simulink library "SimscapeCustomComponents_lib"  (R2025b)
settings: Solver=VariableStepAuto  StartTime=0.0  StopTime=10.0  RelTol=1e-3
undefined symbols (not defined in the file or in its folder): base, baseVdc, capacity, DiscIntNeverNeededParam, ee_sli_rtmsupport, filterInductance, freqeuncy, frequency, gcbh, gflInverter, gfmInverter, iMaxPU, Inertia, initialSOC, plantRating, solar, Ts, ups, Vac, windSystem, windTurbine
libraries: fl_lib x397, nesl_utility x171, eeGeneralControl x85, ee_lib x82, simulink x72, datacenter_lib x68, eeTransforms x38, slpidlib x24, buildingEnergy_lib x20, SimscapeFluids_lib x17, eeSinusoidalMeasurementV2 x8, eePwmGenerator x8
(part 6 of 24)

== system SimscapeCustomComponents_lib/Datacenter/Facilities/Solid State Transformer ==
  note: Cascaded H-Bridge modules with DAB
  note: DAB Control
  note: Rectifier Control
  Constant1 : Constant  Value=dcBusVoltage
  Constant2 : Constant  Value=0
  Converters : Subsystem
      settings: PortSchema="{\"entries\":[{\"content\":{\"sides\":[{\"content\":{\"connectorIds\":[\"In1\",\"In2\",\"LConn1\"]},\"type\":\"ConnectorPlacement.EquallySpacedRectSide\",\"uuid\":\"3c50ecae-d327-4517-ac35-d4ccad8214d6\"},{\"content\":{\"connectorIds\":[\"RConn1\",\"RConn2\",\"Out1\",\"Out2\"],\"side\":\"RIGHT\"},\"type\":\"ConnectorPlacement.EquallySpacedRectSide\",\"uuid\":\"ce483151-8cc4-4e89-a036-44eb982feae5\"},{\"content\":{\"side\":\"TOP\"},\"type\":\"ConnectorPlacement.EquallySpacedRectSide\",\"uuid\":\"39146706-ffb9-4bd3-97cb-72551c78d2ac\"}]},\"type\":\"ConnectorPlacement.EquallySpacedConnector\",\"uuid\":\"8cf16702-94fc-4b9b-91c9-b502d0239b3b\"}],\"packageUris\":[\"http://schema.mathworks.com/mf0/Connector/R2020b\"],\"version\":\"1.0\"}"
  DAB Controller : Subsystem
  DC Voltage Balancing : Subsystem
  Filter & AC measurements : Subsystem
  PFC Rectifier Controller : Subsystem  LoadFcn=%ee_sli_rtmsupport( 'loadfcn', gcbh );  mask(PFC Rectifier Controller (Three-Phase)){Freq=60, L=0.01, BaseImpedance=9.522, KpPLL=15, KiPLL=100, Ts=5e-05, KpVoltage=18, KiVoltage=500, KdVoltage=0, NdVoltage=100, BaseVdc=4400, VoltControlUpperLimit=1, VoltControlLowerLimit=-1, KpdCurrent=10, KidCurrent=200, KddCurrent=0, IdControlUpperLimit=1, IdControlLowerLimit=-1, KpqCurrent=10, KiqCurrent=200, KdqCurrent=0, NdCurrent=100, IqControlUpperLimit=1, IqControlLowerLimit=-1}
      mask prompts: Freq "physmod:ee:library:comments:control:eeConverterControllers:SystemFrequencyHz_MP"; L "physmod:ee:library:comments:control:eeConverterControllers:ACFilterInductanceH_MP"; BaseImpedance "physmod:ee:library:comments:control:eeConverterControllers:ACSideBaseImpedanceOhm_MP"; KpPLL "physmod:ee:library:comments:control:eeConverterControllers:PLLProportionalGain_MP"; KiPLL "physmod:ee:library:comments:control:eeConverterControllers:PLLIntegralGain_MP"; Ts "physmod:ee:library:comments:control:eeConverterControllers:SampleTime1ForInherited_MP"; KpVoltage "physmod:ee:library:comments:control:eeConverterControllers:ProportionalGain_MP"; KiVoltage "physmod:ee:library:comments:control:eeConverterControllers:IntegralGain_MP"; KdVoltage "physmod:ee:library:comments:control:eeConverterControllers:DerivativeGain_MP"; NdVoltage "physmod:ee:library:comments:control:eeConverterControllers:DerivativeControllerFilterCoefficientN_MP"; BaseVdc "physmod:ee:library:comments:control:eeConverterControllers:DCBusBaseVoltageV_MP"; VoltControlUpperLimit "physmod:ee:library:comments:control:eeConverterControllers:ControllerOutputUpperLimitpu_MP"; VoltControlLowerLimit "physmod:ee:library:comments:control:eeConverterControllers:ControllerOutputLowerLimitpu_MP"; KpdCurrent "physmod:ee:library:comments:control:eeConverterControllers:IdProportionalGain_MP"; KidCurrent "physmod:ee:library:comments:control:eeConverterControllers:IdIntegralGain_MP"; KddCurrent "physmod:ee:library:comments:control:eeConverterControllers:IdDerivativeGain_MP"; IdControlUpperLimit "physmod:ee:library:comments:control:eeConverterControllers:IdControllerOutputUpperLimitpu_MP"; IdControlLowerLimit "physmod:ee:library:comments:control:eeConverterControllers:IdControllerOutputLowerLimitpu_MP"; KpqCurrent "physmod:ee:library:comments:control:eeConverterControllers:IqProportionalGain_MP"; KiqCurrent "physmod:ee:library:comments:control:eeConverterControllers:IqIntegralGain_MP"; KdqCurrent "physmod:ee:library:comments:control:eeConverterControllers:IqDerivativeGain_MP"; NdCurrent "physmod:ee:library:comments:control:eeConverterControllers:DerivativeCurrentControllerFilterCoefficientN_MP"; IqControlUpperLimit "physmod:ee:library:comments:control:eeConverterControllers:IqControllerOutputUpperLimitpu_MP"; IqControlLowerLimit "physmod:ee:library:comments:control:eeConverterControllers:IqControllerOutputLowerLimitpu_MP"
      mask help: physmod:ee:library:comments:control:eeConverterControllers:PFCRectifierController_MD
      mask init:
      | ee.mask.initializePFCController(gcb,Ts, Freq, L,BaseImpedance,KpPLL,KiPLL,KpVoltage,KiVoltage,KdVoltage,BaseVdc, NdVoltage,VoltControlUpperLimit,VoltControlLowerLimit,KpdCurrent, KidCurrent, KddCurrent, NdCurrent, IdControlUpperLimit, IdControlLowerLimit, KpqCurrent, KiqCurrent, KdqCurrent, IqControlUpperLimit, IqControlLowerLimit);
      settings: CopyFcn=%ee_sli_rtmsupport( 'copyfcn', gcbh );  DeleteFcn=ee_sli_rtmsupport( 'deletefcn', gcbh );  ModelCloseFcn=ee_sli_rtmsupport( 'modelclosefcn', gcbh );  PostSaveFcn=ee_sli_rtmsupport( 'postsavefcn', gcbh );  PreCopyFcn=ee_sli_rtmsupport( 'precopyfcn', gcbh );  OpenFcn=ee_sli_rtmsupport( 'openfcn', gcbh );  CloseFcn=%ee_sli_rtmsupport( 'closefcn', gcbh );  PreDeleteFcn=ee_sli_rtmsupport( 'predeletefcn', gcbh );
      mask Help: web(nesl_help(gcbh))
      mask DialogControl GeneralTabVal Prompt: physmod:ee:library:comments:control:eeConverterControllers:tab_General
      mask DialogControl Freq Prompt: System frequency (Hz)
      mask DialogControl L Prompt: AC filter inductance (H)
      mask DialogControl BaseImpedance Prompt: AC side base impedance (Ohm)
      mask DialogControl KpPLL Prompt: PLL proportional gain
      mask DialogControl KiPLL Prompt: PLL integral gain
      mask DialogControl Ts Prompt: Sample time (-1 for inherited)
      mask DialogControl VoltageControl Prompt: physmod:ee:library:comments:control:eeConverterControllers:tab_VoltageController
      mask DialogControl KpVoltage Prompt: Proportional gain
      mask DialogControl KiVoltage Prompt: Integral gain
      mask DialogControl KdVoltage Prompt: Derivative gain
      mask DialogControl NdVoltage Prompt: Derivative controller filter coefficient (N)
      mask DialogControl BaseVdc Prompt: DC bus base voltage (V)
      mask DialogControl VoltControlUpperLimit Prompt: Controller output upper limit (pu)
      mask DialogControl VoltControlLowerLimit Prompt: Controller output lower limit (pu)
      mask DialogControl CurrentControl Prompt: physmod:ee:library:comments:control:eeConverterControllers:tab_CurrentController
      mask DialogControl KpdCurrent Prompt: Id proportional gain
      mask DialogControl KidCurrent Prompt: Id integral gain
      mask DialogControl KddCurrent Prompt: Id derivative gain
      mask DialogControl IdControlUpperLimit Prompt: Id controller output upper limit (pu)
      mask DialogControl IdControlLowerLimit Prompt: Id controller output lower limit (pu)
      mask DialogControl KpqCurrent Prompt: Iq proportional gain
      mask DialogControl KiqCurrent Prompt: Iq integral gain
      mask DialogControl KdqCurrent Prompt: Iq derivative gain
      mask DialogControl NdCurrent Prompt: Derivative current controller filter coefficient (N)
      mask DialogControl IqControlUpperLimit Prompt: Iq controller output upper limit (pu)
      mask DialogControl IqControlLowerLimit Prompt: Iq controller output lower limit (pu)
  + : PMIOPort  Side=Right
  - : PMIOPort  Port=2  Side=Right
  ABC : PMIOPort  Port=3  Side=Left
  Out1 : Outport
  wires:
  Constant2/1 -> PFC Rectifier Controller/2(QRef (pu))
  Constant1/1 -> PFC Rectifier Controller/1(VdcRef (V))
  Filter & AC measurements/1(Vabc) -> PFC Rectifier Controller/4(VabcSens (pu))
  Converters/2(VdcMeas) -> PFC Rectifier Controller/3(VdcSens (V))
  Filter & AC measurements/2(Iabc) -> PFC Rectifier Controller/5(IabcSens (pu))
  DC Voltage Balancing/1(mabc) -> Converters/1(mabc)
  Converters/1(Vdc) -> DAB Controller/1(Vdc), DC Voltage Balancing/1(Vdc)
  DAB Controller/1(phi) -> Converters/2(phi)
  PFC Rectifier Controller/1(VabcRef (pu)) -> DC Voltage Balancing/2(VabcRef)
  PFC Rectifier Controller/2(Visualization) -> DAB Controller/2(Vac)
  PFC Rectifier Controller/3(Flag) -> Out1/1
  connections:
  Filter & AC measurements/LConn1 -- ABC/RConn1
  -/RConn1 -- Converters/RConn2
  +/RConn1 -- Converters/RConn1
  Filter & AC measurements/RConn1 -- Converters/LConn1

== system SimscapeCustomComponents_lib/Datacenter/PDU/Cold Plate ==
  Pipe (TL) : fl_lib/Thermal Liquid/Elements/Pipe (TL)  length=pipeLen m  area=pipeArea m^2  Dh=pipeDia m  length_add=pipeLenXtra m  roughness=15e-6 m  Re_lam=2000  Re_tur=4000  shape_factor=64  Nu_lam=3.66  dynamic_compressibility=true  inertia=false  p0=initialP MPa  T0=initialT K  mdot0=0 kg/s  p_nominal=0.101325 MPa  T_nominal=293.15 K
  Thermal Resistance : fl_lib/Thermal/Thermal Elements/Thermal Resistance  resistance=thermalR K/W  T_specify=off  T_priority=None  T=0 K  T_nominal_specify=off  T_nominal_value=1  T_nominal_unit=K  Q_specify=off  Q_priority=None  Q=0 W  Q_nominal_specify=off  Q_nominal_value=1  Q_nominal_unit=W
  A : PMIOPort  Side=Left
  H : PMIOPort  Port=2  Side=Left
  B : PMIOPort  Port=3  Side=Right
  connections:
  Pipe (TL)/RConn1 -- B/RConn1
  Pipe (TL)/LConn1 -- A/RConn1
  Thermal Resistance/RConn1 -- Pipe (TL)/LConn2
  Thermal Resistance/LConn1 -- H/RConn1

== system SimscapeCustomComponents_lib/Datacenter/PDU/PDU Racks ==
  PS Product : fl_lib/Physical Signals/Functions/PS Product
  Server Tray : Subsystem  mask{nGPU=nGPU, gpuTDPperDie=gpuTDPperDie, gpuIdlePower=gpuIdlePower, gpuHBMpower=gpuHBMpower, gpuExponent=gpuExponent, gpuHBMutil=gpuHBMutil, gpuLeakage=gpuLeakage, gpuNominalDieT=gpuNominalDieT, gpuDieThermalC=gpuDieThermalC, gpuHeatSinkR=gpuHeatSinkR, gpuSurfArea=gpuSurfArea, gpuAmbientR=gpuAmbientR, nCPU=nCPU, cpuTDPperSocket=cpuTDPperSocket, cpuIdlePower=cpuIdlePower, cpuExponent=cpuExponent, cpuLeakage=cpuLeakage, cpuNominalDieT=cpuNominalDieT, cpuDieThermalC=cpuDieThermalC, cpuHeatSinkR=cpuHeatSinkR, cpuSurfArea=cpuSurfArea, cpuAmbientR=cpuAmbientR, trayMass=trayMass, trayCp=trayCp, trayThermalR=trayThermalR, initialT=initialT, htc=htc}
      mask prompts: nGPU "Number of GPU (-)"; gpuTDPperDie "GPU TDP per die (W)"; gpuIdlePower "GPU idle power (W)"; gpuHBMpower "HBM power per GPU (W)"; gpuExponent "GPU power utilization exponent (-)"; gpuHBMutil "HBM utilization as fraction of compute utilization (-)"; gpuLeakage "Leakage increase per K above nominal temperature (W/K)"; gpuNominalDieT "Nominal die temperature at TDP (K)"; gpuDieThermalC "GPU die thermal capacitance (J/K)"; gpuHeatSinkR "GPU die-heat-sink thermal resistance (K/W)"; gpuSurfArea "Surface area per die for ambient heat transfer (m^2)"; gpuAmbientR "GPU die-ambient thermal resistance (K/W)"; nCPU "Number of CPU (-)"; cpuTDPperSocket "CPU TDP per socket (W)"; cpuIdlePower "CPU idle power per socket (W)"; cpuExponent "CPU power utilization exponent (-)"; cpuLeakage "Leakage increase per K above nominal temperature (W/K)"; cpuNominalDieT "Nominal die temperature at TDP (K)"; cpuDieThermalC "CPU die thermal capacitance (J/K)"; cpuHeatSinkR "CPU die-heat-sink thermal resistance (K/W)"; cpuSurfArea "Surface area per die for ambient heat transfer (m^2)"; cpuAmbientR "CPU die-ambient thermal resistance (K/W)"; trayMass "Tray mass (kg)"; trayCp "Tray specific heat capacity (J/kg*K)"; trayThermalR "Tray to external thermal resistance (K/W)"; initialT "Initial temperature (K)"; htc "Heat transfer coefficient to ambient (W/m^2.K)"
      settings: CopyFcn=set_param(gcbh,'LinkStatus','none');  PortSchema="{\"entries\":[{\"content\":{\"sides\":[{\"content\":{\"connectorIds\":[\"LConn1\",\"LConn2\",\"LConn3\"]},\"type\":\"ConnectorPlacement.EquallySpacedRectSide\",\"uuid\":\"893f21b9-92d6-433a-96e5-f8193a696c29\"},{\"content\":{\"connectorIds\":[\"RConn1\",\"RConn2\",\"RConn3\"],\"side\":\"RIGHT\"},\"type\":\"ConnectorPlacement.EquallySpacedRectSide\",\"uuid\":\"efd10409-70d8-4a6a-97a2-13f0e6f538e3\"},{\"content\":{\"side\":\"TOP\"},\"type\":\"ConnectorPlacement.EquallySpacedRectSide\",\"uuid\":\"8c9765cd-90e6-46de-916c-606bbb93143e\"},{\"content\":{\"connectorIds\":[\"RConn4\"],\"side\":\"BOTTOM\"},\"type\":\"ConnectorPlacement.EquallySpacedRectSide\",\"uuid\":\"9656b44e-d582-43b0-a7fe-c629821d6c27\"}]},\"type\":\"ConnectorPlacement.EquallySpacedConnector\",\"uuid\":\"add7a682-eb4b-4f46-a5b9-e161ccf96de5\"}],\"packageUris\":[\"http://schema.mathworks.com/mf0/Connector/R2020b\"],\"version\":\"1.0\"}"
      mask Help: web("DocumentationServerTray.html")
      mask DialogControl Container6 Prompt: GPU
      mask DialogControl Container7 Prompt: CPU
      mask DialogControl Container9 Prompt: IT Tray
      mask DialogControl Container8 Prompt: Initial Conditions
      mask Display: image('icon_serverPlate.png');
  TMamb : datacenter_lib/Thermal Multiplier
      settings: InternalSimscapePortConfiguration="{\"Bottom\":[],\"Left\":[{\"id\":\"A\",\"label\":\"A\",\"type\":\"foundation.thermal.thermal\"}],\"Right\":[{\"id\":\"B\",\"label\":\"B\",\"type\":\"foundation.thermal.thermal\"}],\"Top\":[{\"id\":\"Na\",\"label\":\"Na\",\"type\":\"input\"},{\"id\":\"Nb\",\"label\":\"Nb\",\"type\":\"input\"}]}"
  TMcdu : datacenter_lib/Thermal Multiplier
      settings: InternalSimscapePortConfiguration="{\"Bottom\":[],\"Left\":[{\"id\":\"A\",\"label\":\"A\",\"type\":\"foundation.thermal.thermal\"}],\"Right\":[{\"id\":\"B\",\"label\":\"B\",\"type\":\"foundation.thermal.thermal\"}],\"Top\":[{\"id\":\"Na\",\"label\":\"Na\",\"type\":\"input\"},{\"id\":\"Nb\",\"label\":\"Nb\",\"type\":\"input\"}]}"
  nTraysXnRacks : fl_lib/Physical Signals/Sources/PS Constant  constant=nTrays*nRacks
  one : fl_lib/Physical Signals/Sources/PS Constant  constant=1
  U_gpu : PMIOPort  Side=Left
  U_cpu : PMIOPort  Port=2  Side=Left
  Ha : PMIOPort  Port=3  Side=Left
  P : PMIOPort  Port=4  Side=Right
  T_gpu : PMIOPort  Port=5  Side=Right
  T_cpu : PMIOPort  Port=6  Side=Right
  Hc : PMIOPort  Port=7  Side=Right
  connections:
  Server Tray/LConn1 -- U_gpu/RConn1
  TMamb/LConn1 -- Ha/RConn1
  Server Tray/RConn2 -- T_gpu/RConn1
  TMcdu/RConn1 -- Hc/RConn1
  Server Tray/LConn2 -- U_cpu/RConn1
  Server Tray/RConn3 -- T_cpu/RConn1
  one/RConn1 -- TMcdu/LConn3 -- TMamb/LConn2
  Server Tray/RConn4 -- TMcdu/LConn1
  Server Tray/LConn3 -- TMamb/RConn1
  nTraysXnRacks/RConn1 -- PS Product/LConn1 -- TMcdu/LConn2 -- TMamb/LConn3
  Server Tray/RConn1 -- PS Product/LConn2
  PS Product/RConn1 -- P/RConn1

== system SimscapeCustomComponents_lib/Datacenter/PDU/PDU Racks (TL) ==
  FMamb : datacenter_lib/Flow Multiplier
      settings: InternalSimscapePortConfiguration="{\"Bottom\":[],\"Left\":[{\"id\":\"A\",\"label\":\"A\",\"type\":\"foundation.thermal_liquid.thermal_liquid\"}],\"Right\":[{\"id\":\"B\",\"label\":\"B\",\"type\":\"foundation.thermal_liquid.thermal_liquid\"}],\"Top\":[{\"id\":\"Na\",\"label\":\"Na\",\"type\":\"input\"},{\"id\":\"Nb\",\"label\":\"Nb\",\"type\":\"input\"}]}"
  FMcdu : datacenter_lib/Flow Multiplier
      settings: InternalSimscapePortConfiguration="{\"Bottom\":[],\"Left\":[{\"id\":\"A\",\"label\":\"A\",\"type\":\"foundation.thermal_liquid.thermal_liquid\"}],\"Right\":[{\"id\":\"B\",\"label\":\"B\",\"type\":\"foundation.thermal_liquid.thermal_liquid\"}],\"Top\":[{\"id\":\"Na\",\"label\":\"Na\",\"type\":\"input\"},{\"id\":\"Nb\",\"label\":\"Nb\",\"type\":\"input\"}]}"
  PS Product : fl_lib/Physical Signals/Functions/PS Product
  Server Tray (TL) : Subsystem  mask{nGPU=nGPU, gpuTDPperDie=gpuTDPperDie, gpuIdlePower=gpuIdlePower, gpuHBMpower=gpuHBMpower, gpuExponent=gpuExponent, gpuHBMutil=gpuHBMutil, gpuLeakage=gpuLeakage, gpuNominalDieT=gpuNominalDieT, gpuDieThermalC=gpuDieThermalC, gpuHeatSinkR=gpuHeatSinkR, gpuSurfArea=gpuSurfArea, gpuAmbientR=gpuAmbientR, nCPU=nCPU, cpuTDPperSocket=cpuTDPperSocket, cpuIdlePower=cpuIdlePower, cpuExponent=cpuExponent, cpuLeakage=cpuLeakage, cpuNominalDieT=cpuNominalDieT, cpuDieThermalC=cpuDieThermalC, cpuHeatSinkR=cpuHeatSinkR, cpuSurfArea=cpuSurfArea, cpuAmbientR=cpuAmbientR, trayMass=trayMass, trayCp=trayCp, trayThermalR=trayThermalR, pipeLen=pipeLen, pipeArea=pipeArea, pipeDia=pipeDia, pipeLenXtra=pipeLenXtra, thermalKtc=thermalKtc, initialT=initialT, initialP=initialP, htc=htc}
      mask prompts: nGPU "Number of GPU (-)"; gpuTDPperDie "GPU TDP per die (W)"; gpuIdlePower "GPU idle power (W)"; gpuHBMpower "HBM power per GPU (W)"; gpuExponent "GPU power utilization exponent (-)"; gpuHBMutil "HBM utilization as fraction of compute utilization (-)"; gpuLeakage "Leakage increase per K above nominal temperature (W/K)"; gpuNominalDieT "Nominal die temperature at TDP (K)"; gpuDieThermalC "GPU die thermal capacitance (J/K)"; gpuHeatSinkR "GPU die-heat-sink thermal resistance (K/W)"; gpuSurfArea "Surface area per die for ambient heat transfer (m^2)"; gpuAmbientR "GPU die-ambient thermal resistance (K/W)"; nCPU "Number of CPU (-)"; cpuTDPperSocket "CPU TDP per socket (W)"; cpuIdlePower "CPU idle power per socket (W)"; cpuExponent "CPU power utilization exponent (-)"; cpuLeakage "Leakage increase per K above nominal temperature (W/K)"; cpuNominalDieT "Nominal die temperature at TDP (K)"; cpuDieThermalC "CPU die thermal capacitance (J/K)"; cpuHeatSinkR "CPU die-heat-sink thermal resistance (K/W)"; cpuSurfArea "Surface area per die for ambient heat transfer (m^2)"; cpuAmbientR "CPU die-ambient thermal resistance (K/W)"; trayMass "Tray mass (kg)"; trayCp "Tray specific heat capacity (J/kg*K)"; trayThermalR "Tray to external thermal resistance (K/W)"; pipeLen "Cold plate pipe length (m)"; pipeArea "Cold plate pipe cross-sectional area (m^2)"; pipeDia "Cold plate pipe hydraulic diameter (m)"; pipeLenXtra "Cold plate pipe aggregate equivalent length of local resistances (m)"; thermalKtc "Tray to cold plate thermal resistance (K/W)"; initialT "Initial temperature (K)"; initialP "Initial pressure (MPa)"; htc "Heat transfer coefficient to ambient (W/m^2.K)"
      settings: CopyFcn=set_param(gcbh,'LinkStatus','none');  PortSchema="{\"entries\":[{\"content\":{\"sides\":[{\"content\":{\"connectorIds\":[\"LConn1\",\"LConn2\",\"LConn3\"]},\"type\":\"ConnectorPlacement.EquallySpacedRectSide\",\"uuid\":\"d077d73c-67b3-4833-87c7-90e0b4257578\"},{\"content\":{\"connectorIds\":[\"RConn1\",\"RConn2\",\"RConn3\"],\"side\":\"RIGHT\"},\"type\":\"ConnectorPlacement.EquallySpacedRectSide\",\"uuid\":\"5339be23-611e-4862-9a5e-dd4e1a595af9\"},{\"content\":{\"side\":\"TOP\"},\"type\":\"ConnectorPlacement.EquallySpacedRectSide\",\"uuid\":\"df4f00c7-722c-4787-b527-29bc4d99befa\"},{\"content\":{\"connectorIds\":[\"RConn4\",\"RConn5\"],\"side\":\"BOTTOM\"},\"type\":\"ConnectorPlacement.EquallySpacedRectSide\",\"uuid\":\"45f86463-19b5-41c3-bb79-cbbcfbdd4a59\"}]},\"type\":\"ConnectorPlacement.EquallySpacedConnector\",\"uuid\":\"da9ddc4c-7978-4ef3-ba33-dfd55a606f60\"}],\"packageUris\":[\"http://schema.mathworks.com/mf0/Connector/R2020b\"],\"version\":\"1.0\"}"
      mask Help: web("DocumentationServerTrayTL.html")
      mask DialogControl Container6 Prompt: GPU
      mask DialogControl Container7 Prompt: CPU
      mask DialogControl Container9 Prompt: IT Tray
      mask DialogControl Container8 Prompt: Initial Conditions
      mask Display: image('icon_serverPlateTL.png');
  TMamb : datacenter_lib/Thermal Multiplier
      settings: InternalSimscapePortConfiguration="{\"Bottom\":[],\"Left\":[{\"id\":\"A\",\"label\":\"A\",\"type\":\"foundation.thermal.thermal\"}],\"Right\":[{\"id\":\"B\",\"label\":\"B\",\"type\":\"foundation.thermal.thermal\"}],\"Top\":[{\"id\":\"Na\",\"label\":\"Na\",\"type\":\"input\"},{\"id\":\"Nb\",\"label\":\"Nb\",\"type\":\"input\"}]}"
  nTraysXnRacks : fl_lib/Physical Signals/Sources/PS Constant  constant=nTrays*nRacks
  one : fl_lib/Physical Signals/Sources/PS Constant  constant=1
  U_gpu : PMIOPort  Side=Left
  U_cpu : PMIOPort  Port=2  Side=Left
  Ha : PMIOPort  Port=3  Side=Left
  P : PMIOPort  Port=4  Side=Right
  T_gpu : PMIOPort  Port=5  Side=Right
  T_cpu : PMIOPort  Port=6  Side=Right
  A : PMIOPort  Port=7  Side=Right
  B : PMIOPort  Port=8  Side=Right
  connections:
  Server Tray (TL)/RConn1 -- PS Product/LConn2
  Server Tray (TL)/LConn2 -- U_cpu/RConn1
  Server Tray (TL)/RConn3 -- T_cpu/RConn1
  Server Tray (TL)/RConn2 -- T_gpu/RConn1
  FMcdu/LConn1 -- Server Tray (TL)/RConn5
  FMamb/LConn1 -- Server Tray (TL)/RConn4
  PS Product/LConn1 -- TMamb/LConn3 -- FMcdu/LConn2 -- FMamb/LConn2 -- nTraysXnRacks/RConn1
  FMamb/LConn3 -- FMcdu/LConn3 -- TMamb/LConn2 -- one/RConn1
  FMcdu/RConn1 -- B/RConn1
  FMamb/RConn1 -- A/RConn1
  PS Product/RConn1 -- P/RConn1
  Server Tray (TL)/LConn1 -- U_gpu/RConn1
  TMamb/RConn1 -- Server Tray (TL)/LConn3
  TMamb/LConn1 -- Ha/RConn1

== system SimscapeCustomComponents_lib/Datacenter/PDU/Server Tray ==
  AmbCPU : fl_lib/Thermal/Thermal Elements/Convective Heat Transfer  thermal_type=foundation.enum.constant_variable.constant  area=cpuSurfArea*nCPU m^2  heat_tr_coeff=htc W/(K*m^2)  min_heat_tr_coeff=1e-3 W/(K*m^2)  T_specify=off  T_priority=None  T=0 K  T_nominal_specify=off  T_nominal_value=1  T_nominal_unit=K  Q_specify=off  Q_priority=None  Q=0 W  Q_nominal_specify=off  Q_nominal_value=1  Q_nominal_unit=W
  AmbGPU : fl_lib/Thermal/Thermal Elements/Convective Heat Transfer  thermal_type=foundation.enum.constant_variable.constant  area=gpuSurfArea*nGPU m^2  heat_tr_coeff=htc W/(K*m^2)  min_heat_tr_coeff=1e-3 W/(K*m^2)  T_specify=off  T_priority=None  T=0 K  T_nominal_specify=off  T_nominal_value=1  T_nominal_unit=K  Q_specify=off  Q_priority=None  Q=0 W  Q_nominal_specify=off  Q_nominal_value=1  Q_nominal_unit=W
  PS Add : fl_lib/Physical Signals/Functions/PS Add
  Server Chip CPU : datacenter_lib/Server Chip  processorType=ProcessorType.CPU  numGPUs=4  numCPUs=nCPU  gpuTDP=1200 W  gpuIdlePower=300 W  gpuPowerExponent=1.4  hbmPowPerGPU=80 W  hbmUtilizationFrac=0.7  cpuTDP=cpuTDPperSocket W  cpuIdlePower=cpuIdlePower W  cpuPowerExponent=cpuExponent  PleakageCoeff=cpuLeakage W/K  chipTnominal=cpuNominalDieT K  chipCth=cpuDieThermalC J/K  T_specify=on  T_priority=High  T=initialT K  T_nominal_specify=off  T_nominal_value=1  T_nominal_unit=K  Q_specify=off  Q_priority=None  Q=0 W  Q_nominal_specify=off  Q_nominal_value=1  Q_nominal_unit=W
      settings: InternalSimscapePortConfiguration="{\"Bottom\":[{\"id\":\"H\",\"label\":\"H\",\"type\":\"foundation.thermal.thermal\"}],\"Left\":[{\"id\":\"U\",\"label\":\"U\",\"type\":\"input\"}],\"Right\":[{\"id\":\"Pow\",\"label\":\"P\",\"type\":\"output\"},{\"id\":\"Tchip\",\"label\":\"T\",\"type\":\"output\"}],\"Top\":[]}"
  Server Chip GPU : datacenter_lib/Server Chip  processorType=ProcessorType.GPU  numGPUs=nGPU  numCPUs=nCPU  gpuTDP=gpuTDPperDie W  gpuIdlePower=gpuIdlePower W  gpuPowerExponent=gpuExponent  hbmPowPerGPU=gpuHBMpower W  hbmUtilizationFrac=gpuHBMutil  cpuTDP=cpuTDPperSocket W  cpuIdlePower=cpuIdlePower W  cpuPowerExponent=1.1  PleakageCoeff=gpuLeakage W/K  chipTnominal=gpuNominalDieT K  chipCth=gpuDieThermalC J/K  T_specify=on  T_priority=High  T=initialT K  T_nominal_specify=off  T_nominal_value=1  T_nominal_unit=K  Q_specify=off  Q_priority=None  Q=0 W  Q_nominal_specify=off  Q_nominal_value=1  Q_nominal_unit=W
      settings: InternalSimscapePortConfiguration="{\"Bottom\":[{\"id\":\"H\",\"label\":\"H\",\"type\":\"foundation.thermal.thermal\"}],\"Left\":[{\"id\":\"U\",\"label\":\"U\",\"type\":\"input\"}],\"Right\":[{\"id\":\"Pow\",\"label\":\"P\",\"type\":\"output\"},{\"id\":\"Tchip\",\"label\":\"T\",\"type\":\"output\"}],\"Top\":[]}"
  TR_CPU_Amb : fl_lib/Thermal/Thermal Elements/Thermal Resistance  resistance=cpuAmbientR/nCPU K/W  T_specify=off  T_priority=None  T=0 K  T_nominal_specify=off  T_nominal_value=1  T_nominal_unit=K  Q_specify=off  Q_priority=None  Q=0 W  Q_nominal_specify=off  Q_nominal_value=1  Q_nominal_unit=W
  TR_CPU_substrate : fl_lib/Thermal/Thermal Elements/Thermal Resistance  resistance=cpuHeatSinkR/nCPU K/W  T_specify=off  T_priority=None  T=0 K  T_nominal_specify=off  T_nominal_value=1  T_nominal_unit=K  Q_specify=off  Q_priority=None  Q=0 W  Q_nominal_specify=off  Q_nominal_value=1  Q_nominal_unit=W
  TR_GPU_Amb : fl_lib/Thermal/Thermal Elements/Thermal Resistance  resistance=gpuAmbientR/nGPU K/W  T_specify=off  T_priority=None  T=0 K  T_nominal_specify=off  T_nominal_value=1  T_nominal_unit=K  Q_specify=off  Q_priority=None  Q=0 W  Q_nominal_specify=off  Q_nominal_value=1  Q_nominal_unit=W
  TR_GPU_substrate : fl_lib/Thermal/Thermal Elements/Thermal Resistance  resistance=gpuHeatSinkR/nGPU K/W  T_specify=off  T_priority=None  T=0 K  T_nominal_specify=off  T_nominal_value=1  T_nominal_unit=K  Q_specify=off  Q_priority=None  Q=0 W  Q_nominal_specify=off  Q_nominal_value=1  Q_nominal_unit=W
  TR_Tray_Amb : fl_lib/Thermal/Thermal Elements/Thermal Resistance  resistance=trayThermalR K/W  T_specify=off  T_priority=None  T=0 K  T_nominal_specify=off  T_nominal_value=1  T_nominal_unit=K  Q_specify=off  Q_priority=None  Q=0 W  Q_nominal_specify=off  Q_nominal_value=1  Q_nominal_unit=W
  Tray Thermal Mass : fl_lib/Thermal/Thermal Elements/Thermal Mass  mass_type=foundation.enum.constant_variable.constant  mass=trayMass kg  sp_heat=trayCp J/(K*kg)  mass_min=1e-6 kg  num_ports=foundation.enum.numPorts2.two  m_specify=off  m_priority=High  m=1 kg  m_nominal_specify=off  m_nominal_value=1  m_nominal_unit=kg  T_specify=on  T_priority=High  T=initialT K  T_nominal_specify=off  T_nominal_value=1  T_nominal_unit=K  Q_specify=off  Q_priority=None  Q=0 W  Q_nominal_specify=off  Q_nominal_value=1  Q_nominal_unit=W
      settings: InternalSimscapePortConfiguration="{\"Bottom\":[],\"Left\":[{\"id\":\"M\",\"label\":\"\",\"type\":\"foundation.thermal.thermal\"}],\"Right\":[{\"id\":\"N\",\"label\":\"\",\"type\":\"foundation.thermal.thermal\"}],\"Top\":[]}"
  U_gpu : PMIOPort  Side=Left
  U_cpu : PMIOPort  Port=2  Side=Left
  P : PMIOPort  Port=3  Side=Right
  T_gpu : PMIOPort  Port=4  Side=Right
  T_cpu : PMIOPort  Port=5  Side=Right
  Hc : PMIOPort  Port=6  Side=Right
  Ha : PMIOPort  Port=7  Side=Left
  connections:
  Tray Thermal Mass/LConn1 -- TR_GPU_substrate/RConn1 -- TR_CPU_substrate/RConn1
  Server Chip GPU/RConn2 -- T_gpu/RConn1
  TR_CPU_substrate/LConn1 -- TR_CPU_Amb/LConn1 -- Server Chip CPU/RConn3
  TR_GPU_Amb/RConn1 -- Server Chip GPU/RConn3 -- TR_GPU_substrate/LConn1
  TR_Tray_Amb/LConn1 -- Tray Thermal Mass/RConn1
  Server Chip GPU/LConn1 -- U_gpu/RConn1
  Server Chip CPU/LConn1 -- U_cpu/RConn1
  Server Chip CPU/RConn2 -- T_cpu/RConn1
  TR_Tray_Amb/RConn1 -- Hc/RConn1
  AmbGPU/LConn1 -- TR_GPU_Amb/LConn1
  AmbCPU/RConn1 -- AmbGPU/RConn1 -- Ha/RConn1
  P/RConn1 -- PS Add/RConn1
  PS Add/LConn1 -- Server Chip GPU/RConn1
  PS Add/LConn2 -- Server Chip CPU/RConn1
  AmbCPU/LConn1 -- TR_CPU_Amb/RConn1

== system SimscapeCustomComponents_lib/Datacenter/PDU/Server Tray (TL) ==
  Cold Plate : Subsystem  mask{pipeLen=pipeLen, pipeArea=pipeArea, pipeDia=pipeDia, pipeLenXtra=pipeLenXtra, thermalR=thermalKtc, initialT=initialT, initialP=initialP}
      mask prompts: pipeLen "Cold plate pipe length (m)"; pipeArea "Pipe cross-section area (m^2)"; pipeDia "Pipe hydraulic diameter (m)"; pipeLenXtra "Aggregate equivalent length of local resistances (m)"; thermalR "IT tray to cold plate thermal resistance (K/W)"; initialT "Initial temperature (K)"; initialP "Initial pressure (MPa)"
      settings: CopyFcn=set_param(gcbh,'LinkStatus','none');  PortSchema="{\"entries\":[{\"content\":{\"sides\":[{\"content\":{\"connectorIds\":[\"LConn1\"]},\"type\":\"ConnectorPlacement.EquallySpacedRectSide\",\"uuid\":\"8838d57f-01eb-4279-bd1c-25d25bcf5ace\"},{\"content\":{\"connectorIds\":[\"RConn1\"],\"side\":\"RIGHT\"},\"type\":\"ConnectorPlacement.EquallySpacedRectSide\",\"uuid\":\"56ae8252-1580-44dd-87b9-8c427bc34f49\"},{\"content\":{\"connectorIds\":[\"LConn2\"],\"side\":\"TOP\"},\"type\":\"ConnectorPlacement.EquallySpacedRectSide\",\"uuid\":\"52c6abaa-a3e9-4948-a21c-7378e8bd6fd9\"}]},\"type\":\"ConnectorPlacement.EquallySpacedConnector\",\"uuid\":\"7eb709cb-ec6a-4cc7-adbc-64cff18012b9\"}],\"packageUris\":[\"http://schema.mathworks.com/mf0/Connector/R2020b\"],\"version\":\"1.0\"}"
      mask Help: web("DocumentationColdPlate.html")
      mask DialogControl Container4 Prompt: Cold Plate
      mask DialogControl Container5 Prompt: Initial Conditions
      mask Display: image('icon_coldplate.png');
  Server Tray : Subsystem  mask{nGPU=nGPU, gpuTDPperDie=gpuTDPperDie, gpuIdlePower=gpuIdlePower, gpuHBMpower=gpuHBMpower, gpuExponent=gpuExponent, gpuHBMutil=gpuHBMutil, gpuLeakage=gpuLeakage, gpuNominalDieT=gpuLeakage, gpuDieThermalC=gpuDieThermalC, gpuHeatSinkR=gpuHeatSinkR, gpuSurfArea=gpuSurfArea, gpuAmbientR=gpuAmbientR, nCPU=nCPU, cpuTDPperSocket=cpuTDPperSocket, cpuIdlePower=cpuIdlePower, cpuExponent=cpuExponent, cpuLeakage=cpuLeakage, cpuNominalDieT=cpuNominalDieT, cpuDieThermalC=cpuDieThermalC, cpuHeatSinkR=cpuHeatSinkR, cpuSurfArea=cpuSurfArea, cpuAmbientR=cpuAmbientR, trayMass=trayMass, trayCp=trayCp, trayThermalR=trayThermalR, initialT=initialT, htc=htc}
      mask prompts: nGPU "Number of GPU (-)"; gpuTDPperDie "GPU TDP per die (W)"; gpuIdlePower "GPU idle power (W)"; gpuHBMpower "HBM power per GPU (W)"; gpuExponent "GPU power utilization exponent (-)"; gpuHBMutil "HBM utilization as fraction of compute utilization (-)"; gpuLeakage "Leakage increase per K above nominal temperature (W/K)"; gpuNominalDieT "Nominal die temperature at TDP (K)"; gpuDieThermalC "GPU die thermal capacitance (J/K)"; gpuHeatSinkR "GPU die-heat-sink thermal resistance (K/W)"; gpuSurfArea "Surface area per die for ambient heat transfer (m^2)"; gpuAmbientR "GPU die-ambient thermal resistance (K/W)"; nCPU "Number of CPU (-)"; cpuTDPperSocket "CPU TDP per socket (W)"; cpuIdlePower "CPU idle power per socket (W)"; cpuExponent "CPU power utilization exponent (-)"; cpuLeakage "Leakage increase per K above nominal temperature (W/K)"; cpuNominalDieT "Nominal die temperature at TDP (K)"; cpuDieThermalC "CPU die thermal capacitance (J/K)"; cpuHeatSinkR "CPU die-heat-sink thermal resistance (K/W)"; cpuSurfArea "Surface area per die for ambient heat transfer (m^2)"; cpuAmbientR "CPU die-ambient thermal resistance (K/W)"; trayMass "Tray mass (kg)"; trayCp "Tray specific heat capacity (J/kg*K)"; trayThermalR "Tray to external thermal resistance (K/W)"; initialT "Initial temperature (K)"; htc "Heat transfer coefficient to ambient (W/m^2.K)"
      settings: CopyFcn=set_param(gcbh,'LinkStatus','none');  PortSchema="{\"entries\":[{\"content\":{\"sides\":[{\"content\":{\"connectorIds\":[\"LConn1\",\"LConn2\",\"LConn3\"]},\"type\":\"ConnectorPlacement.EquallySpacedRectSide\",\"uuid\":\"893f21b9-92d6-433a-96e5-f8193a696c29\"},{\"content\":{\"connectorIds\":[\"RConn1\",\"RConn2\",\"RConn3\"],\"side\":\"RIGHT\"},\"type\":\"ConnectorPlacement.EquallySpacedRectSide\",\"uuid\":\"efd10409-70d8-4a6a-97a2-13f0e6f538e3\"},{\"content\":{\"side\":\"TOP\"},\"type\":\"ConnectorPlacement.EquallySpacedRectSide\",\"uuid\":\"8c9765cd-90e6-46de-916c-606bbb93143e\"},{\"content\":{\"connectorIds\":[\"RConn4\"],\"side\":\"BOTTOM\"},\"type\":\"ConnectorPlacement.EquallySpacedRectSide\",\"uuid\":\"9656b44e-d582-43b0-a7fe-c629821d6c27\"}]},\"type\":\"ConnectorPlacement.EquallySpacedConnector\",\"uuid\":\"add7a682-eb4b-4f46-a5b9-e161ccf96de5\"}],\"packageUris\":[\"http://schema.mathworks.com/mf0/Connector/R2020b\"],\"version\":\"1.0\"}"
      mask Help: web("DocumentationServerTray.html")
      mask DialogControl Container6 Prompt: GPU
      mask DialogControl Container7 Prompt: CPU
      mask DialogControl Container9 Prompt: IT Tray
      mask DialogControl Container8 Prompt: Initial Conditions
      mask Display: image('icon_serverPlate.png');
  U_gpu : PMIOPort  Side=Left
  U_cpu : PMIOPort  Port=2  Side=Left
  Ha : PMIOPort  Port=3  Side=Left
  P : PMIOPort  Port=4  Side=Right
  T_gpu : PMIOPort  Port=5  Side=Right
  T_cpu : PMIOPort  Port=6  Side=Right
  A : PMIOPort  Port=7  Side=Right
  B : PMIOPort  Port=8  Side=Right
  connections:
  Cold Plate/LConn2 -- Server Tray/RConn4
  Server Tray/LConn3 -- Ha/RConn1
  Server Tray/LConn1 -- U_gpu/RConn1
  Server Tray/LConn2 -- U_cpu/RConn1
  Cold Plate/LConn1 -- A/RConn1
  Cold Plate/RConn1 -- B/RConn1
  Server Tray/RConn1 -- P/RConn1
  Server Tray/RConn3 -- T_cpu/RConn1
  Server Tray/RConn2 -- T_gpu/RConn1

== system SimscapeCustomComponents_lib/Microgrid and Renewables/Control/BESS ==
  Grid Following Control : Subsystem  VariantControl=Grid Following  mask(Grid Following Controller){mp=0.0001, mv=0.02, P=Real power, MVA=480e3, frequency=50, zbase=0.002, L=1e-3, Imax=1.2, Td=1e-3, Kpic=0.1, Kiic=1, Kd=0}
      mask prompts: mp "Real power droop cofficient"; mv "Reactive power droop cofficient"; P "Priority mode"; MVA "Base Power (V*A)"; frequency "Frequency (Hz)"; zbase "Base Impedance (Ohm)"; L "Filter Inductance (H)"; Imax "Inverter current limit (pu)"; Td "Sensor time delay (s)"; Kpic "Proportional gain"; Kiic "Integral gain"; Kd "Derevative gain"
      mask help: This block implements a Grid Following control strategy where the BESS synchronizes with an existing grid voltage and frequency. Ideal for systems where the grid is strong and the BESS acts as a power source following grid conditions.
      settings: CopyFcn=set_param(gcb,'LinkStatus','none');
      mask Help: web('GFLController.html')
      mask TypeOptions P: Real power  | Reactive power
      mask DialogControl Container4 Prompt: General
      mask DialogControl Container5 Prompt: Current Controller
      mask Display: image('gridfollowing2_2_9_7_2_1.png');
  Grid Forming Control : Subsystem  VariantControl=Grid Forming  mask(Grid Forming Controller){power=2.2e6, girdLineVoltage=690, powerFreq=50, dcBusVoltage=1500, measSampleTime=1e-3, powerControl=Virtual Synchronous Machine, activePowerSampleTime=1e-3, droopSlope=gfmInverter.droopControl.freqSlopeMp*350, droopT1=gfmInverter.droopControl.T1, droopT2=gfmInverter.droopControl.T2, droopTC=gfmInverter.droopControl.lpfTimeConst, vsmPmeasFilterTC=1e-3, vsmFreqDroop=1, vsmInertiaTC=10, vsmDampingConst=1, dampingPowerMaxLimit=0.9, dampingPowerMinLimit=-0.9, freqMeasTimeConst=1e-3, freqOption=Constant Frequency Reference, voltreference=1, QVoltFilterTC=1e-3, QVoltDroop=10, currentLimit=Current Limiting, maxSatCurrentLimit=1.2, maxVICurrentLimit=gfmInverter.currentLimit.viCurrentLimit, ctLimitVirtualImp=gfmInverter.currentLimit.virImpResistanceCoeff, ctLimitXbyR=gfmInverter.currentLimit.virImpXbyR, ctLimitDelayTime=0.1, currentSatTime=gfmInverter.currentLimit.satCurrentRunTime, currentVITimeConst=gfmInverter.currentLimit.viFilterTimeConst, voltControlTs=5e-5, vdPGain=0.1, VdIGain=1, VdMaxCt=1.2, VdMinCt=0.8, VqPGain=0.1, VqIGain=1, VqMaxCt=1.2, VqMinCt=0.8, vdvqLPFTimeConst=1e-3, currentControlTs=5e-5, filterInductance=1e-3, IdPGain=0.1, IdIGain=1, IqPGain=0.1, IqIGain=1}
      mask prompts: power "Grid forming converter power (VA)"; girdLineVoltage "Grid line voltage (V)"; powerFreq "Grid frequency (Hz)"; dcBusVoltage "DC bus voltage"; measSampleTime "Measurement sample time"; powerControl "Active Power Control"; activePowerSampleTime "Sample time (s)"; droopSlope "Power droop slope (pu, Hz/W)"; droopT1 "Lead-Lag numerator time constant (s)"; droopT2 "Lead-Lag denominator time constant (s)"; droopTC "Filter cut-off time constant (s)"; vsmPmeasFilterTC "Power measurement filter time constant (s)"; vsmFreqDroop "Frequency droop (pu,  W/Hz)"; vsmInertiaTC "Inertia constant M (pu)"; vsmDampingConst "Damping constant (pu/Hz)"; dampingPowerMaxLimit "Damping power maximum limit (pu)"; dampingPowerMinLimit "Damping power minimum limit (pu)"; freqMeasTimeConst "Frequency measurement time constant (s)"; freqOption "Damping power fequency option"; voltreference "Voltage reference value (pu)"; QVoltFilterTC "Power measurement filter time constant (s)"; QVoltDroop "Voltage droop (pu, V/VAR)"; currentLimit "Current limiting method"; maxSatCurrentLimit "Maximum current saturation (pu)"; maxVICurrentLimit "Maximum virtual impedance current (pu)"; ctLimitVirtualImp "Virtual impedance coefficient (pu.Ohm/pu.A)"; ctLimitXbyR "Virtual X/R ratio"; ctLimitDelayTime "Maximum current delay time (s)"; currentSatTime "Current limiting run time (s)"; currentVITimeConst "Filter time constant (s)"; voltControlTs "Controller sample time (s)"; vdPGain "Vd proportional gain"; VdIGain "Vd integral gain"; VdMaxCt "Vd maximum current limit (A)"; VdMinCt "Vd minimum current limit (A)"; VqPGain "Vq proportional gain"; VqIGain "Vq integral gain"; VqMaxCt "Vq maximum current limit (A)"; VqMinCt "Vq minimum current limit (A)"; vdvqLPFTimeConst "Voltage measurement filter time constant (s)"; currentControlTs "Controller sample time (s)"; filterInductance "Filter inductance (H)"; IdPGain "Id proportional gain"; IdIGain "Id integral gain"; IqPGain "Iq proportional gain"; IqIGain "Iq integral gain"
      mask help: This block implements the grid forming controller with fault ride through capability. Input to the controller are active and reactive power reference in per unit and the sensed three-phase phase current in amphere and phase voltage in volts.
      mask init:
      | powerChoice = get_param(gcb,'powerControl');
      | currentChoice = get_param(gcb,'currentLimit');
      | 
      | powerloc = [gcb, '/Power Control/ActivePowerControl']; 
      | currentloc = [gcb, '/Current Limiting/CurrentLimitingMethod'];
      | freqLoc = [gcb,'/Power Control/ActivePowerControl/vsmControl/Damping Frequency'];
      | 
      | switch powerChoice
      |     case 'Virtual Synchronous Machine'
      |         set_param(powerloc, 'LabelModeActiveChoice', 'vsm');
      |         dampingFreqChoice = get_param(gcb,'freqOption');
      |         if strcmp(dampingFreqChoice,'Use Grid Frequency Measurement')
      |             set_param(freqLoc, 'LabelModeActiveChoice', 'freqMeas');
      |         else
      |             set_param(freqLoc, 'LabelModeActiveChoice', 'constFreq');
      |         end
      |     case 'Droop Control'
      |          set_param(powerloc, 'LabelModeActiveChoice', 'droop');
      |    otherwise
      |         disp('Choose proper active power control method')
      | end
      | switch currentChoice
      |     case 'Virtual Impedance'
      |           set_param(currentloc, 'LabelModeActiveChoice', 'virimp');
      |     case 'Current Limiting'
      |          set_param(currentloc, 'LabelModeActiveChoice', 'ctSat');
      |     case 'Combining Virtual Impedance and Current Limiting'
      |             set_param(currentloc, 'LabelModeActiveChoice', 'both');
      |     otherwise
      |         disp('Choose proper current limiting method')
      | end
      settings: CopyFcn=set_param(gcb,'LinkStatus','none');
      mask Help: web('GFMController.html')
      mask TypeOptions powerControl: Virtual Synchronous Machine | Droop Control
      mask Callback powerControl:
      | h = Simulink.Mask.get(gcb);
      | slectedActivePowerControl=get_param(gcb,'powerControl');
      | %slectedActivePowerControl = h.Parameters(find(string({h.Parameters.Name}) == 'powerControl')).Value;
      | switch slectedActivePowerControl
      |     case 'Virtual Synchronous Machine'
      |         h.Parameters(find(string({h.Parameters.Name}) == 'droopSlope')).Visible = 'off';
      |         h.Parameters(find(string({h.Parameters.Name}) == 'droopTC')).Visible = 'off';
      |         h.Parameters(find(string({h.Parameters.Name}) == 'droopT1')).Visible = 'off';
      |         h.Parameters(find(string({h.Parameters.Name}) == 'droopT2')).Visible = 'off';
      |         h.Parameters(find(string({h.Parameters.Name}) == 'vsmPmeasFilterTC')).Visible = 'on';
      |         h.Parameters(find(string({h.Parameters.Name}) == 'vsmFreqDroop')).Visible = 'on';
      |         h.Parameters(find(string({h.Parameters.Name}) == 'vsmInertiaTC')).Visible = 'on';
      |         h.Parameters(find(string({h.Parameters.Name}) == 'vsmDampingConst')).Visible = 'on';
      |         h.Parameters(find(string({h.Parameters.Name}) == 'dampingPowerMaxLimit')).Visible = 'on';
      |         h.Parameters(find(string({h.Parameters.Name}) == 'dampingPowerMinLimit')).Visible = 'on';
      |         h.Parameters(find(string({h.Parameters.Name}) == 'freqOption')).Visible = 'on';
      |         h.Parameters(find(string({h.Parameters.Name}) == 'freqMeasTimeConst')).Visible = 'on';
      |     case 'Droop Control'
      |         h.Parameters(find(string({h.Parameters.Name}) == 'droopSlope')).Visible = 'on';
      |         h.Parameters(find(string({h.Parameters.Name}) == 'droopTC')).Visible = 'on';
      |         h.Parameters(find(string({h.Parameters.Name}) == 'droopT1')).Visible = 'on';
      |         h.Parameters(find(string({h.Parameters.Name}) == 'droopT2')).Visible = 'on';
      |         h.Parameters(find(string({h.Parameters.Name}) == 'vsmPmeasFilterTC')).Visible = 'off';
      |         h.Parameters(find(string({h.Parameters.Name}) == 'vsmFreqDroop')).Visible = 'off';
      |         h.Parameters(find(string({h.Parameters.Name}) == 'vsmInertiaTC')).Visible = 'off';
      |         h.Parameters(find(string({h.Parameters.Name}) == 'vsmDampingConst')).Visible = 'off';
      |         h.Parameters(find(string({h.Parameters.Name}) == 'dampingPowerMaxLimit')).Visible = 'off';
      |         h.Parameters(find(string({h.Parameters.Name}) == 'dampingPowerMinLimit')).Visible = 'off';
      |         h.Parameters(find(string({h.Parameters.Name}) == 'freqOption')).Visible = 'off';
      |         h.Parameters(find(string({h.Parameters.Name}) == 'freqMeasTimeConst')).Visible = 'on';
      | 
      |     otherwise
      |         disp('Choose proper active power control method')
      | end
      mask TypeOptions freqOption: Use Grid Frequency Measurement | Constant Frequency Reference
      mask TypeOptions currentLimit: Virtual Impedance | Current Limiting | Combining Virtual Impedance and Current Limiting
      mask Callback currentLimit:
      | currentLimit = 1;
      | h = Simulink.Mask.get(gcb);
      | currentLimitControl=get_param(gcb,'currentLimit');
      | %slectedActivePowerControl = h.Parameters(find(string({h.Parameters.Name}) == 'powerControl')).Value;
      | switch currentLimitControl
      |     case 'Virtual Impedance'
      |         h.Parameters(find(string({h.Parameters.Name}) == 'maxVICurrentLimit')).Visible = 'on';
      |         h.Parameters(find(string({h.Parameters.Name}) == 'ctLimitVirtualImp')).Visible = 'on';
      |         h.Parameters(find(string({h.Parameters.Name}) == 'ctLimitXbyR')).Visible = 'on';
      |         h.Parameters(find(string({h.Parameters.Name}) == 'maxSatCurrentLimit')).Visible = 'off';
      |         h.Parameters(find(string({h.Parameters.Name}) == 'ctLimitDelayTime')).Visible = 'off';
      |         h.Parameters(find(string({h.Parameters.Name}) == 'currentSatTime')).Visible = 'off';
      |         h.Parameters(find(string({h.Parameters.Name}) == 'currentVITimeConst')).Visible = 'on';
      | 
      | 
      |     case 'Current Limiting'
      |         h.Parameters(find(string({h.Parameters.Name}) == 'maxVICurrentLimit')).Visible = 'off';
      |         h.Parameters(find(string({h.Parameters.Name}) == 'ctLimitVirtualImp')).Visible = 'off';
      |         h.Parameters(find(string({h.Parameters.Name}) == 'ctLimitXbyR')).Visible = 'off';
      |         h.Parameters(find(string({h.Parameters.Name}) == 'maxSatCurrentLimit')).Visible = 'on';
      |         h.Parameters(find(string({h.Parameters.Name}) == 'ctLimitDelayTime')).Visible = 'on';
      |         h.Parameters(find(string({h.Parameters.Name}) == 'currentSatTime')).Visible = 'off';
      |         h.Parameters(find(string({h.Parameters.Name}) == 'currentVITimeConst')).Visible = 'off';
      | 
      |     case 'Combining Virtual Impedance and Current Limiting'
      |         h.Parameters(find(string({h.Parameters.Name}) == 'maxVICurrentLimit')).Visible = 'on';
      |         h.Parameters(find(string({h.Parameters.Name}) == 'ctLimitVirtualImp')).Visible = 'on';
      |         h.Parameters(find(string({h.Parameters.Name}) == 'ctLimitXbyR')).Visible = 'on';
      |         h.Parameters(find(string({h.Parameters.Name}) == 'maxSatCurrentLimit')).Visible = 'on';
      |         h.Parameters(find(string({h.Parameters.Name}) == 'ctLimitDelayTime')).Visible = 'off';
      |         h.Parameters(find(string({h.Parameters.Name}) == 'currentSatTime')).Visible = 'on';
      |         h.Parameters(find(string({h.Parameters.Name}) == 'currentVITimeConst')).Visible = 'on';
      | 
      |     otherwise
      |         disp('Choose proper current limiting method')
      | end
      mask DialogControl ParameterGroupVar Prompt: Grid Forming Control Parameters
      mask DialogControl Container8 Prompt: Grid-forming Converter Specification
      mask DialogControl Pcontrolgrp Prompt: Active Power Controller Parameters
      mask DialogControl QcontrolGrp Prompt: Reactive Power Controller Parameters
      mask DialogControl faultRideThroughGrp Prompt: Fault Ride Through Parameters
      mask DialogControl voltControlgrp Prompt: Voltage Controller Parameters
      mask DialogControl Container15currentContGrp Prompt: Current Controller Parameters
      mask Display: image('gfmGridFormingConverterVSM1_1_7_7_2.png');

== system SimscapeCustomComponents_lib/Microgrid and Renewables/Control/Generator ==
  "Governor and Prime Mover " : Subsystem  mask(Governor and Prime Mover){pu_speed_reference=1, droop_percentage=10, pu_load_reference_setpoint=1, T_G=0.01, T_CH=0.001, base_torque=18143, pu_torque0=18143}
      mask prompts: pu_speed_reference "Speed reference, (pu)"; droop_percentage "Percentage droop, (%)"; pu_load_reference_setpoint "Load reference setpoint, (pu)"; T_G "Time constant of governor, (s)"; T_CH "Time constant of main inlet volumes and steam chest, (s)"; base_torque "Base torque, (N*m)"; pu_torque0 "Initial torque, (pu)"
      mask help:
      | Implements a synchronous machine governor and prime mover. The prime mover is a non-reheat steam turbine.
      |
      | The input to the block is a per-unit synchronous machine measurement vector.
      |
      | R and C are mechanical rotational ports.
      settings: CopyFcn=set_param(gcbh,'LinkStatus','none');

== system SimscapeCustomComponents_lib/Microgrid and Renewables/Control/Microgrid ==
  Black Start : Subsystem  mask(BlackStart){referenceFrequency=50, controllerBlackStart=2, voltageLevel1=0.3, voltageLevel2=0.3, voltageLevel3=0.2, delayLevel1=2, delayLevel2=2, delayLevel3=2}
      mask prompts: referenceFrequency "Reference Frequency"; controllerBlackStart "Black Start Time"; voltageLevel1 "Level1"; voltageLevel2 "Level2"; voltageLevel3 "Level3"; delayLevel1 "Delay1"; delayLevel2 "Delay2"; delayLevel3 "Delay3"
      mask help: This block implements the black start logic in the microgrid
      settings: CopyFcn=set_param(gcbh,'LinkStatus','none')
      mask Help: web('BlackStart.html')
      mask DialogControl Container4 Prompt: General
      mask DialogControl Container5 Prompt: Voltage Levels
      mask DialogControl Container6 Prompt: Time Delay
  PlannedIslanding : Subsystem  mask(PlannedIslanding){KpPPlannedIsland=1, KiPPlannedIsland=5, ZeroActivePowerThreshold=0.1, KpQPlannedIsland=1, KiQPlannedIsland=5, ZeroReactivePowerThreshold=0.5}
      mask prompts: KpPPlannedIsland "Proportional Gain"; KiPPlannedIsland "Integral Gain"; ZeroActivePowerThreshold "Threshold"; KpQPlannedIsland "Proportional Gain"; KiQPlannedIsland "Integral Gain"; ZeroReactivePowerThreshold "Threshold"
      mask help: This block enables the microgrid to island from the grid in a planned manner by reducing the active and reactive power from the grid
      settings: CopyFcn=set_param(gcbh,'LinkStatus','none');
      mask Help: web('PlannedIslanding.html')
      mask DialogControl Container4 Prompt: Active Power
      mask DialogControl Container5 Prompt: Reactive Power
  Resynchronization : Subsystem  mask(Resynchronization){GridFrequency=50, KpVolResynch=0.1, KiVolResynch=0.01, VoltageThreshold=0.05, kDroop=0, KpFreResynch=0.1, KiFreResynch=0.01, FrequencyThreshold=0.05, KpAngResynch=0.1, KiAngResynch=0.01, AngleThreshold=0.05}
      mask prompts: GridFrequency "Grid Frequency"; KpVolResynch "Proportional Gain"; KiVolResynch "Integral Gain"; kDroop "Voltage Droop"; KpFreResynch "Proportional Gain"; KiFreResynch "Integral Gain"; KpAngResynch "Proportional Gain"; KiAngResynch "Integral Gain"
      mask help: This block enables the microgrid to reconnect with the grid if the voltage, frequency and angle of the islanded microgrid matches to the grid with certain threshold
      settings: CopyFcn=set_param(gcbh,'LinkStatus','none');
      mask Help: web('Resynchronization.html')
      mask DialogControl Container4 Prompt: General
      mask DialogControl Container6 Prompt: Voltage
      mask DialogControl Container5 Prompt: Frequency
      mask DialogControl Container7 Prompt: Angle
